simulink model "four_bots_CNN_DSM_7"  (R2018b)
settings: Solver=ode5  StartTime=0.0  StopTime=20.0  FixedStep=0.0002  RelTol=1e-3
(part 1 of 2)
settings Model: Creator=a1752760  LastModifiedBy=a1752760

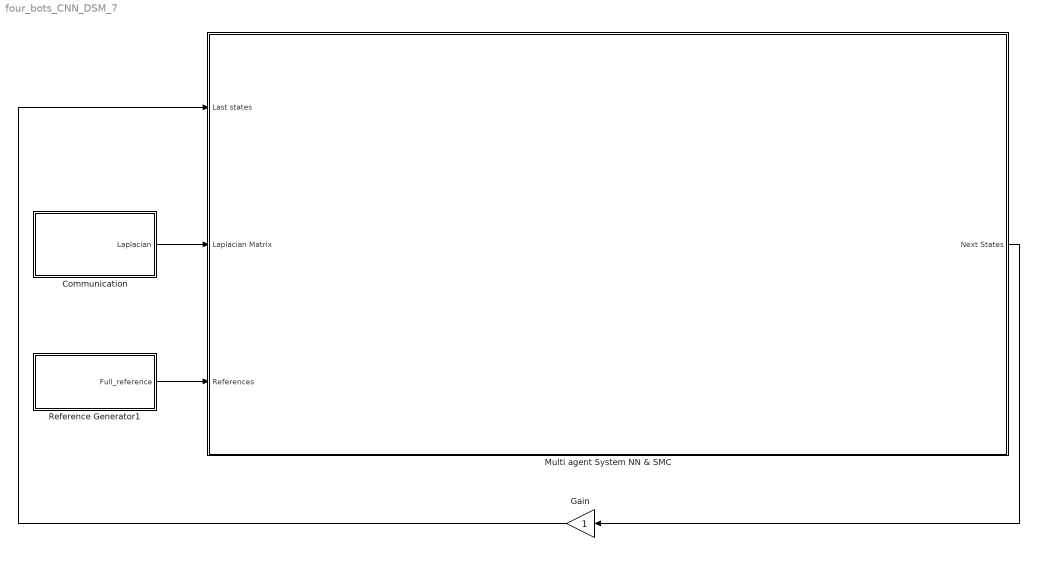
== system four_bots_CNN_DSM_7 ==
  Communication : Subsystem
  Gain : Gain
  Multi agent System NN & SMC : Subsystem
  Reference Generator1 : Subsystem
  wires:
  Multi agent System NN & SMC/1(Next States) -> Gain/1
  Communication/1(Laplacian) -> Multi agent System NN & SMC/2(Laplacian Matrix)
  Reference Generator1/1(Full_reference) -> Multi agent System NN & SMC/3("References ")
  Gain/1 -> Multi agent System NN & SMC/1(Last states)

== system four_bots_CNN_DSM_7/Communication ==
  Add : Sum
  Communication Topology : Constant  Value=[2,-1,0,-1;-1,2,-1,0;0,-1,2,-1;-1,0,-1,2]  VectorParams1D=off
  Constant : Constant  Value=2  VectorParams1D=off
  Product : Product
  Reference Feeding : Constant  Value=[1,0,0,0;0,1,0,0;0,0,1,0;0,0,0,1]  VectorParams1D=off
  Laplacian : Outport
  wires:
  Constant/1 -> Product/2
  Reference Feeding/1 -> Product/1
  Communication Topology/1 -> Add/1
  Product/1 -> Add/2
  Add/1 -> Laplacian/1

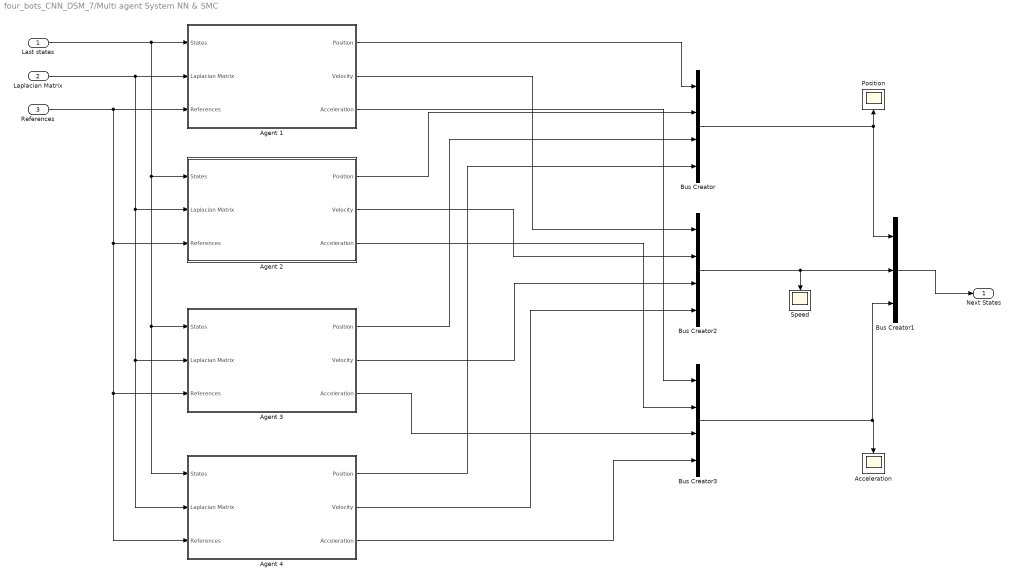
== system four_bots_CNN_DSM_7/Multi agent System NN & SMC ==
  Last states : Inport
  Laplacian Matrix : Inport  Port=2
  "References " : Inport  Port=3
  Acceleration : Scope
  "Agent 1 " : Subsystem
  Agent 2 : Subsystem
  Agent 3 : Subsystem
  Agent 4 : Subsystem
  Bus Creator : BusCreator  Inputs=4
  Bus Creator1 : BusCreator  Inputs=3
  Bus Creator2 : BusCreator  Inputs=4
  Bus Creator3 : BusCreator  Inputs=4
  Position : Scope
  Speed : Scope
  Next States : Outport
  wires:
  Bus Creator1/1 -> Next States/1
  Last states/1 -> Agent 4/1(States), Agent 3/1(States), Agent 2/1(States), "Agent 1 "/1(States)
  Laplacian Matrix/1 -> Agent 4/2(Laplacian Matrix), Agent 3/2(Laplacian Matrix), Agent 2/2(Laplacian Matrix), "Agent 1 "/2(Laplacian Matrix)
  "References "/1 -> Agent 4/3("References "), Agent 3/3("References "), Agent 2/3("References "), "Agent 1 "/3("References ")
  "Agent 1 "/1(Position) -> Bus Creator/1
  Agent 2/1(Position) -> Bus Creator/2
  Agent 3/1(Position) -> Bus Creator/3
  Agent 4/1(Position) -> Bus Creator/4
  "Agent 1 "/2(Velocity) -> Bus Creator2/1
  Agent 2/2(Velocity) -> Bus Creator2/2
  Agent 3/2(Velocity) -> Bus Creator2/3
  Agent 4/2(Velocity) -> Bus Creator2/4
  "Agent 1 "/3(Acceleration) -> Bus Creator3/1
  Agent 2/3(Acceleration) -> Bus Creator3/2
  Agent 3/3(Acceleration) -> Bus Creator3/3
  Agent 4/3(Acceleration) -> Bus Creator3/4
  Bus Creator/1 -> Bus Creator1/1, Position/1
  Bus Creator2/1 -> Speed/1, Bus Creator1/2
  Bus Creator3/1 -> Bus Creator1/3, Acceleration/1

== system four_bots_CNN_DSM_7/Reference Generator1 ==
  Acceleration reference : MATLAB Function  TreatAsAtomicUnit=on
  Acceleration_dot Reference : MATLAB Function  TreatAsAtomicUnit=on
  Acceleration_dot_ref : Scope
  Acceleration_ref : Scope
  Bus Creator1 : BusCreator  Inputs=4
  Clock : Clock
  Position Reference : MATLAB Function  TreatAsAtomicUnit=on
  Position_ref : Scope
  Speed Reference : MATLAB Function  TreatAsAtomicUnit=on
  Speed_ref : Scope
  Full_reference : Outport
  wires:
  Clock/1 -> Acceleration_dot Reference/1(t), Acceleration reference/1(t), Speed Reference/1(t), Position Reference/1(t)
  Position Reference/1(x1d) -> Position_ref/1, Bus Creator1/1
  Speed Reference/1(x2d) -> Speed_ref/1, Bus Creator1/2
  Acceleration reference/1(x2d_dot) -> Acceleration_ref/1, Bus Creator1/3
  Acceleration_dot Reference/1(x2ddot) -> Acceleration_dot_ref/1, Bus Creator1/4
  Bus Creator1/1 -> Full_reference/1

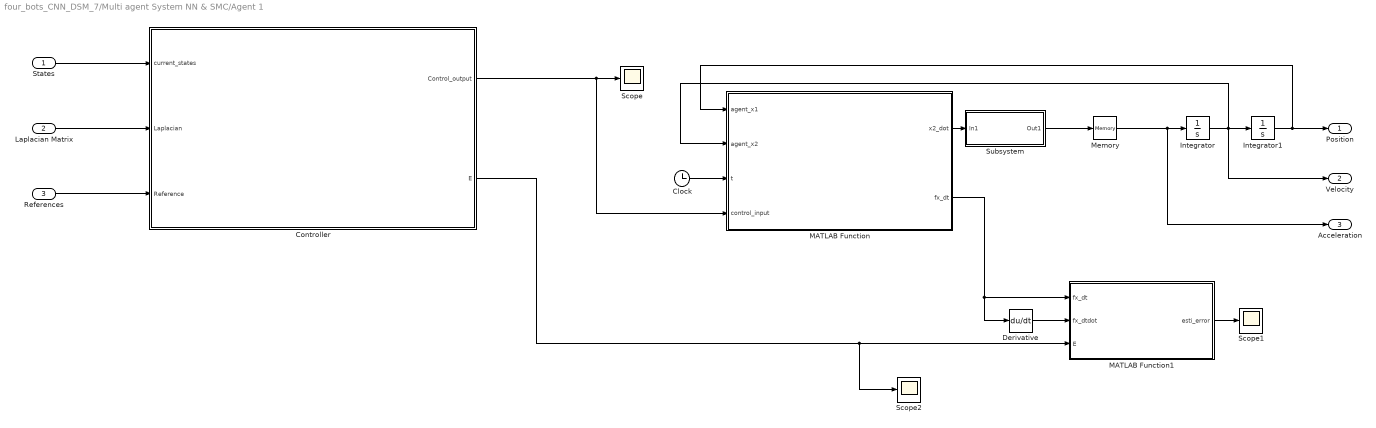
== system four_bots_CNN_DSM_7/Multi agent System NN & SMC/Agent 1  ==
  States : Inport
  Laplacian Matrix : Inport  Port=2
  "References " : Inport  Port=3
  Clock : Clock
  "Controller " : Subsystem
  Derivative : Derivative
  Integrator : Integrator  InitialCondition=[0;0;0]  ContinuousStateAttributes='speed'
  Integrator1 : Integrator  Tag=Position_x1  InitialCondition=[2;-1.5;-pi/3]  ContinuousStateAttributes='position'
  MATLAB Function : MATLAB Function  TreatAsAtomicUnit=on
  MATLAB Function1 : MATLAB Function  TreatAsAtomicUnit=on
  Memory : Memory  InitialCondition=[0;0;0]  LinearizeMemory=on
  Scope : Scope
  Scope1 : Scope
  Scope2 : Scope
  Subsystem : Subsystem
  Position : Outport
  Velocity : Outport  Port=2
  Acceleration : Outport  Port=3
  wires:
  MATLAB Function/2(fx_dt) -> MATLAB Function1/1(fx_dt), Derivative/1
  Integrator/1 -> Velocity/1, Integrator1/1, MATLAB Function/2(agent_x2)
  Integrator1/1 -> Position/1, MATLAB Function/1(agent_x1)
  MATLAB Function/1(x2_dot) -> Subsystem/1(In1)
  Subsystem/1(Out1) -> Memory/1
  States/1 -> "Controller "/1(current_states)
  Laplacian Matrix/1 -> "Controller "/2(Laplacian)
  "References "/1 -> "Controller "/3(Reference)
  "Controller "/1(Control_output) -> MATLAB Function/4(control_input), Scope/1
  Clock/1 -> MATLAB Function/3(t)
  Derivative/1 -> MATLAB Function1/2(fx_dtdot)
  "Controller "/2(E) -> Scope2/1, MATLAB Function1/3(E)
  MATLAB Function1/1(esti_error) -> Scope1/1
  Memory/1 -> Acceleration/1, Integrator/1

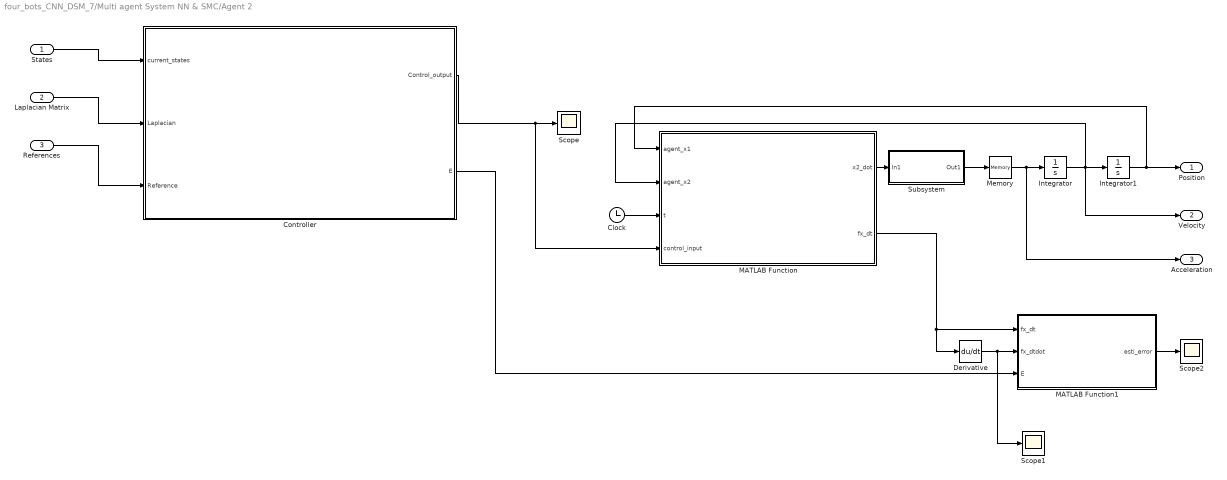
== system four_bots_CNN_DSM_7/Multi agent System NN & SMC/Agent 2 ==
  States : Inport
  Laplacian Matrix : Inport  Port=2
  "References " : Inport  Port=3
  Clock : Clock
  "Controller " : Subsystem
  Derivative : Derivative
  Integrator : Integrator  InitialCondition=[0;0;0]  ContinuousStateAttributes='speed'
  Integrator1 : Integrator  Tag=Position_x1  InitialCondition=[-1;1.5;pi/4]  ContinuousStateAttributes='position'
  MATLAB Function : MATLAB Function  TreatAsAtomicUnit=on
  MATLAB Function1 : MATLAB Function  TreatAsAtomicUnit=on
  Memory : Memory  InitialCondition=[0;0;0]  LinearizeMemory=on
  Scope : Scope
  Scope1 : Scope
  Scope2 : Scope
  Subsystem : Subsystem
  Position : Outport
  Velocity : Outport  Port=2
  Acceleration : Outport  Port=3
  wires:
  Integrator/1 -> Velocity/1, Integrator1/1, MATLAB Function/2(agent_x2)
  Integrator1/1 -> Position/1, MATLAB Function/1(agent_x1)
  MATLAB Function/1(x2_dot) -> Subsystem/1(In1)
  Subsystem/1(Out1) -> Memory/1
  States/1 -> "Controller "/1(current_states)
  Laplacian Matrix/1 -> "Controller "/2(Laplacian)
  "References "/1 -> "Controller "/3(Reference)
  "Controller "/1(Control_output) -> MATLAB Function/4(control_input), Scope/1
  "Controller "/2(E) -> MATLAB Function1/3(E)
  MATLAB Function1/1(esti_error) -> Scope2/1
  Derivative/1 -> Scope1/1, MATLAB Function1/2(fx_dtdot)
  MATLAB Function/2(fx_dt) -> MATLAB Function1/1(fx_dt), Derivative/1
  Clock/1 -> MATLAB Function/3(t)
  Memory/1 -> Acceleration/1, Integrator/1

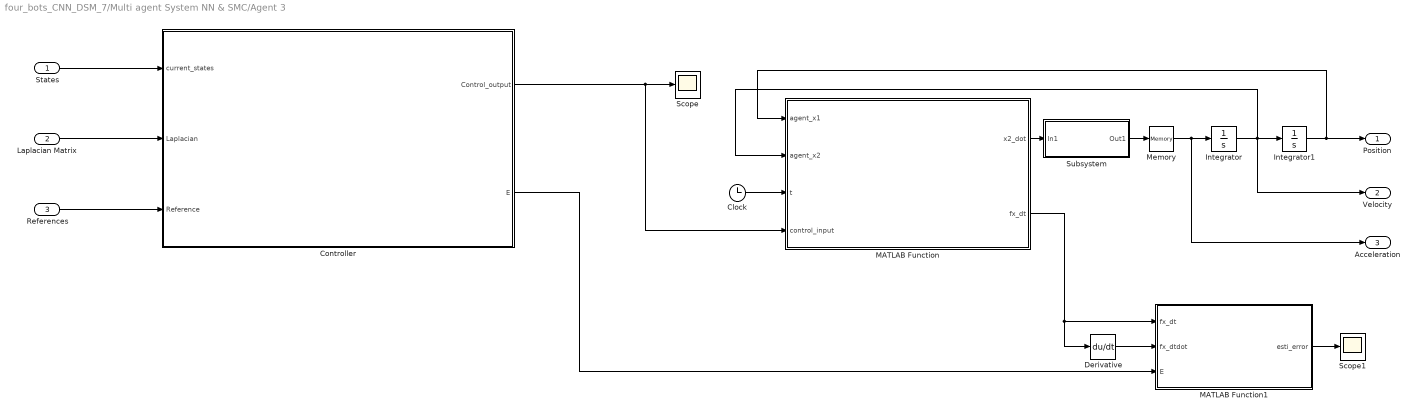
== system four_bots_CNN_DSM_7/Multi agent System NN & SMC/Agent 3 ==
  States : Inport
  Laplacian Matrix : Inport  Port=2
  "References " : Inport  Port=3
  Clock : Clock
  "Controller " : Subsystem
  Derivative : Derivative
  Integrator : Integrator  InitialCondition=[0;0;0]  ContinuousStateAttributes='speed'
  Integrator1 : Integrator  Tag=Position_x1  InitialCondition=[-3.5;1.5;-pi/6]  ContinuousStateAttributes='position'
  MATLAB Function : MATLAB Function  TreatAsAtomicUnit=on
  MATLAB Function1 : MATLAB Function  TreatAsAtomicUnit=on
  Memory : Memory  InitialCondition=[0;0;0]  LinearizeMemory=on
  Scope : Scope
  Scope1 : Scope
  Subsystem : Subsystem
  Position : Outport
  Velocity : Outport  Port=2
  Acceleration : Outport  Port=3
  wires:
  MATLAB Function/2(fx_dt) -> MATLAB Function1/1(fx_dt), Derivative/1
  Integrator/1 -> Velocity/1, Integrator1/1, MATLAB Function/2(agent_x2)
  Integrator1/1 -> Position/1, MATLAB Function/1(agent_x1)
  MATLAB Function/1(x2_dot) -> Subsystem/1(In1)
  Subsystem/1(Out1) -> Memory/1
  States/1 -> "Controller "/1(current_states)
  Laplacian Matrix/1 -> "Controller "/2(Laplacian)
  "References "/1 -> "Controller "/3(Reference)
  "Controller "/1(Control_output) -> MATLAB Function/4(control_input), Scope/1
  Clock/1 -> MATLAB Function/3(t)
  Derivative/1 -> MATLAB Function1/2(fx_dtdot)
  "Controller "/2(E) -> MATLAB Function1/3(E)
  MATLAB Function1/1(esti_error) -> Scope1/1
  Memory/1 -> Acceleration/1, Integrator/1

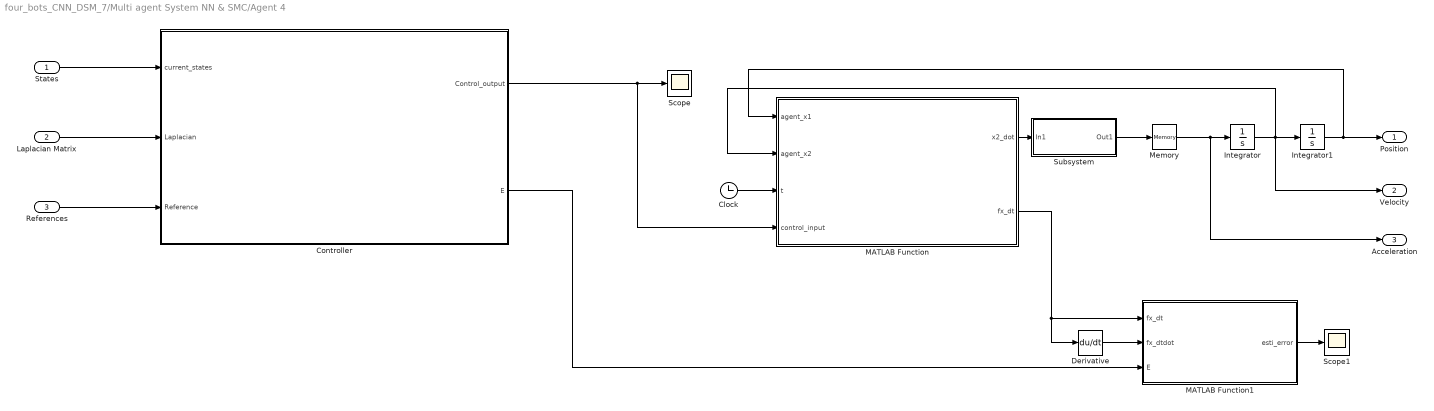
== system four_bots_CNN_DSM_7/Multi agent System NN & SMC/Agent 4 ==
  States : Inport
  Laplacian Matrix : Inport  Port=2
  "References " : Inport  Port=3
  Clock : Clock
  "Controller " : Subsystem
  Derivative : Derivative
  Integrator : Integrator  InitialCondition=[0;0;0]  ContinuousStateAttributes='speed'
  Integrator1 : Integrator  Tag=Position_x1  InitialCondition=[1.8;-3.3;pi/6]  ContinuousStateAttributes='position'
  MATLAB Function : MATLAB Function  TreatAsAtomicUnit=on
  MATLAB Function1 : MATLAB Function  TreatAsAtomicUnit=on
  Memory : Memory  InitialCondition=[0;0;0]  LinearizeMemory=on
  Scope : Scope
  Scope1 : Scope
  Subsystem : Subsystem
  Position : Outport
  Velocity : Outport  Port=2
  Acceleration : Outport  Port=3
  wires:
  MATLAB Function/2(fx_dt) -> MATLAB Function1/1(fx_dt), Derivative/1
  Integrator/1 -> Velocity/1, Integrator1/1, MATLAB Function/2(agent_x2)
  Integrator1/1 -> Position/1, MATLAB Function/1(agent_x1)
  MATLAB Function/1(x2_dot) -> Subsystem/1(In1)
  Subsystem/1(Out1) -> Memory/1
  States/1 -> "Controller "/1(current_states)
  Laplacian Matrix/1 -> "Controller "/2(Laplacian)
  "References "/1 -> "Controller "/3(Reference)
  "Controller "/1(Control_output) -> MATLAB Function/4(control_input), Scope/1
  Clock/1 -> MATLAB Function/3(t)
  Derivative/1 -> MATLAB Function1/2(fx_dtdot)
  "Controller "/2(E) -> MATLAB Function1/3(E)
  MATLAB Function1/1(esti_error) -> Scope1/1
  Memory/1 -> Acceleration/1, Integrator/1

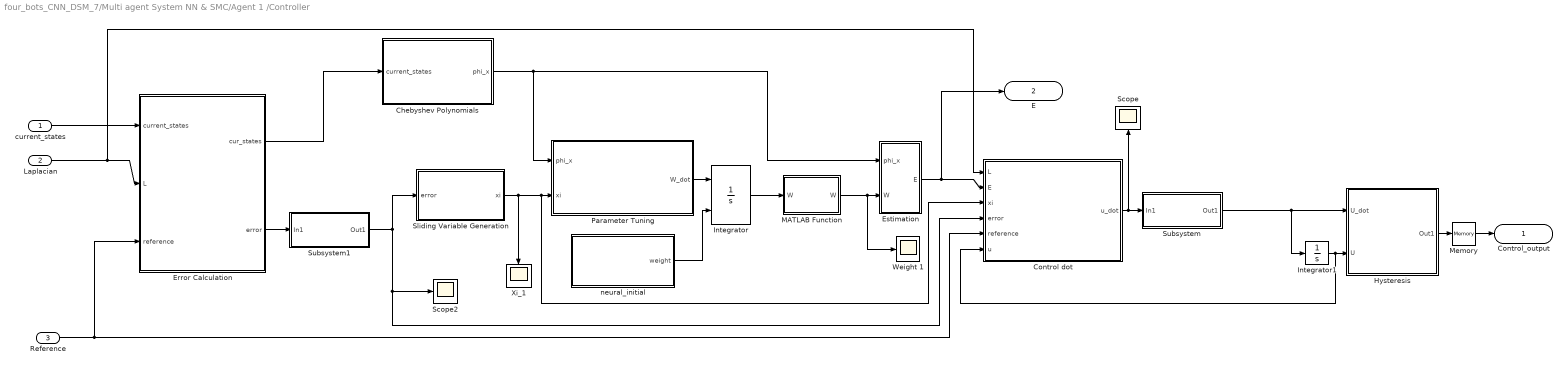
== system four_bots_CNN_DSM_7/Multi agent System NN & SMC/Agent 1 /Controller  ==
  current_states : Inport
  Laplacian : Inport  Port=2
  Reference : Inport  Port=3
  Chebyshev Polynomials : MATLAB Function  TreatAsAtomicUnit=on
  Control dot : MATLAB Function  TreatAsAtomicUnit=on
  Error Calculation : MATLAB Function  TreatAsAtomicUnit=on
  Estimation : MATLAB Function  TreatAsAtomicUnit=on
  Hysteresis : Subsystem
  Integrator : Integrator  InitialConditionSource=external  InitialCondition=[0 0 0]'  UpperSaturationLimit=200  LowerSaturationLimit=-200  ContinuousStateAttributes='Neural_weights'
  Integrator1 : Integrator  InitialCondition=[0;0;0]  UpperSaturationLimit=200  LowerSaturationLimit=-200  ContinuousStateAttributes='Control_output'
  MATLAB Function : MATLAB Function  TreatAsAtomicUnit=on
  Memory : Memory  InitialCondition=[0;0;0]  LinearizeMemory=on
  Parameter Tuning : MATLAB Function  TreatAsAtomicUnit=on
  Scope : Scope
  Scope2 : Scope
  Sliding Variable Generation : MATLAB Function  TreatAsAtomicUnit=on
  Subsystem : Subsystem
  Subsystem1 : Subsystem
  Weight 1 : Scope
  Xi_1 : Scope
  neural_initial : MATLAB Function  TreatAsAtomicUnit=on
  Control_output : Outport
  E : Outport  Port=2
  wires:
  current_states/1 -> Error Calculation/1(current_states)
  Reference/1 -> Error Calculation/3(reference), Control dot/5(reference)
  Sliding Variable Generation/1(xi) -> Xi_1/1, Control dot/3(xi), Parameter Tuning/2(xi)
  Chebyshev Polynomials/1(phi_x) -> Estimation/1(phi_x), Parameter Tuning/1(phi_x)
  Parameter Tuning/1(W_dot) -> Integrator/1
  neural_initial/1(weight) -> Integrator/2
  Integrator/1 -> MATLAB Function/1("W ")
  Estimation/1(E) -> E/1, Control dot/2(E)
  Control dot/1(u_dot) -> Subsystem/1(In1), Scope/1
  Error Calculation/2(error) -> Subsystem1/1(In1)
  Subsystem1/1(Out1) -> Sliding Variable Generation/1(error), Control dot/4(error), Scope2/1
  Integrator1/1 -> Hysteresis/2(U), Control dot/6(u)
  Laplacian/1 -> Control dot/1(L), Error Calculation/2(L)
  Error Calculation/1(cur_states) -> Chebyshev Polynomials/1(current_states)
  Hysteresis/1(Out1) -> Memory/1
  Subsystem/1(Out1) -> Integrator1/1, Hysteresis/1(U_dot)
  Memory/1 -> Control_output/1
  MATLAB Function/1(W) -> Weight 1/1, Estimation/2(W)

== system four_bots_CNN_DSM_7/Multi agent System NN & SMC/Agent 1 /Subsystem ==
  In1 : Inport
  Clock : Clock
  Constant : Constant  Value=[0;0;0]
  Scope3 : Scope
  Switch : Switch  Criteria=u2 > Threshold  Threshold=0.01
  Out1 : Outport
  wires:
  Constant/1 -> Switch/3
  In1/1 -> Switch/1
  Switch/1 -> Out1/1, Scope3/1
  Clock/1 -> Switch/2

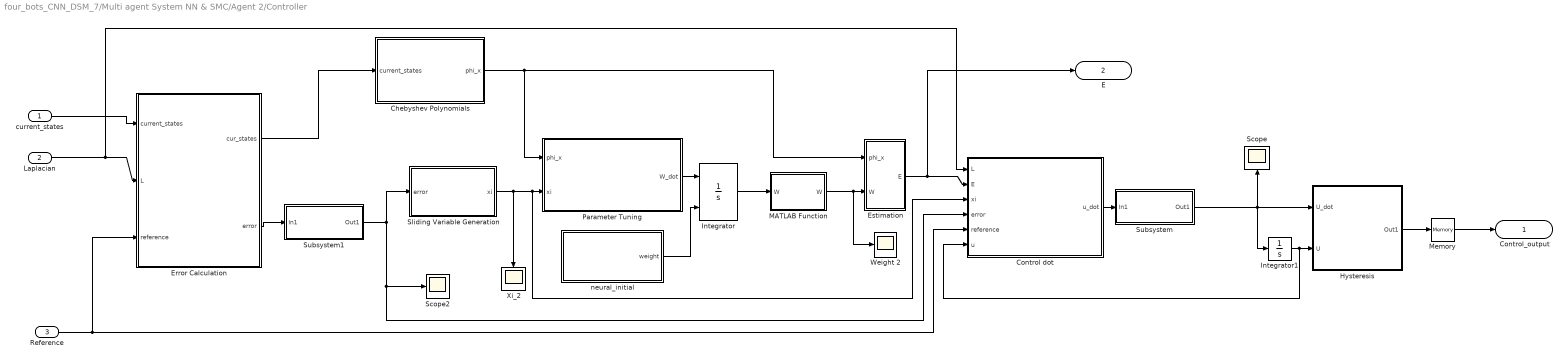
== system four_bots_CNN_DSM_7/Multi agent System NN & SMC/Agent 2/Controller  ==
  current_states : Inport
  Laplacian : Inport  Port=2
  Reference : Inport  Port=3
  Chebyshev Polynomials : MATLAB Function  TreatAsAtomicUnit=on
  Control dot : MATLAB Function  TreatAsAtomicUnit=on
  Error Calculation : MATLAB Function  TreatAsAtomicUnit=on
  Estimation : MATLAB Function  TreatAsAtomicUnit=on
  Hysteresis : Subsystem
  Integrator : Integrator  InitialConditionSource=external  InitialCondition=[0 0 0]'  UpperSaturationLimit=200  LowerSaturationLimit=-200  ContinuousStateAttributes='Neural_weights'
  Integrator1 : Integrator  InitialCondition=[0;0;0]  UpperSaturationLimit=200  LowerSaturationLimit=-200  ContinuousStateAttributes='Control_output'
  MATLAB Function : MATLAB Function  TreatAsAtomicUnit=on
  Memory : Memory  InitialCondition=[0;0;0]  LinearizeMemory=on
  Parameter Tuning : MATLAB Function  TreatAsAtomicUnit=on
  Scope : Scope
  Scope2 : Scope
  Sliding Variable Generation : MATLAB Function  TreatAsAtomicUnit=on
  Subsystem : Subsystem
  Subsystem1 : Subsystem
  Weight 2 : Scope
  Xi_2 : Scope
  neural_initial : MATLAB Function  TreatAsAtomicUnit=on
  Control_output : Outport
  E : Outport  Port=2
  wires:
  current_states/1 -> Error Calculation/1(current_states)
  Reference/1 -> Error Calculation/3(reference), Control dot/5(reference)
  Sliding Variable Generation/1(xi) -> Xi_2/1, Control dot/3(xi), Parameter Tuning/2(xi)
  Chebyshev Polynomials/1(phi_x) -> Estimation/1(phi_x), Parameter Tuning/1(phi_x)
  Parameter Tuning/1(W_dot) -> Integrator/1
  neural_initial/1(weight) -> Integrator/2
  Integrator/1 -> MATLAB Function/1("W ")
  Estimation/1(E) -> E/1, Control dot/2(E)
  Control dot/1(u_dot) -> Subsystem/1(In1)
  Error Calculation/2(error) -> Subsystem1/1(In1)
  Subsystem1/1(Out1) -> Sliding Variable Generation/1(error), Control dot/4(error), Scope2/1
  Integrator1/1 -> Hysteresis/2(U), Control dot/6(u)
  Laplacian/1 -> Control dot/1(L), Error Calculation/2(L)
  Error Calculation/1(cur_states) -> Chebyshev Polynomials/1(current_states)
  Hysteresis/1(Out1) -> Memory/1
  Subsystem/1(Out1) -> Integrator1/1, Scope/1, Hysteresis/1(U_dot)
  Memory/1 -> Control_output/1
  MATLAB Function/1(W) -> Weight 2/1, Estimation/2(W)

== system four_bots_CNN_DSM_7/Multi agent System NN & SMC/Agent 2/Subsystem ==
  In1 : Inport
  Clock : Clock
  Constant : Constant  Value=[0;0;0]
  Scope3 : Scope
  Switch : Switch  Criteria=u2 > Threshold  Threshold=0.01
  Out1 : Outport
  wires:
  Constant/1 -> Switch/3
  In1/1 -> Switch/1
  Switch/1 -> Out1/1, Scope3/1
  Clock/1 -> Switch/2

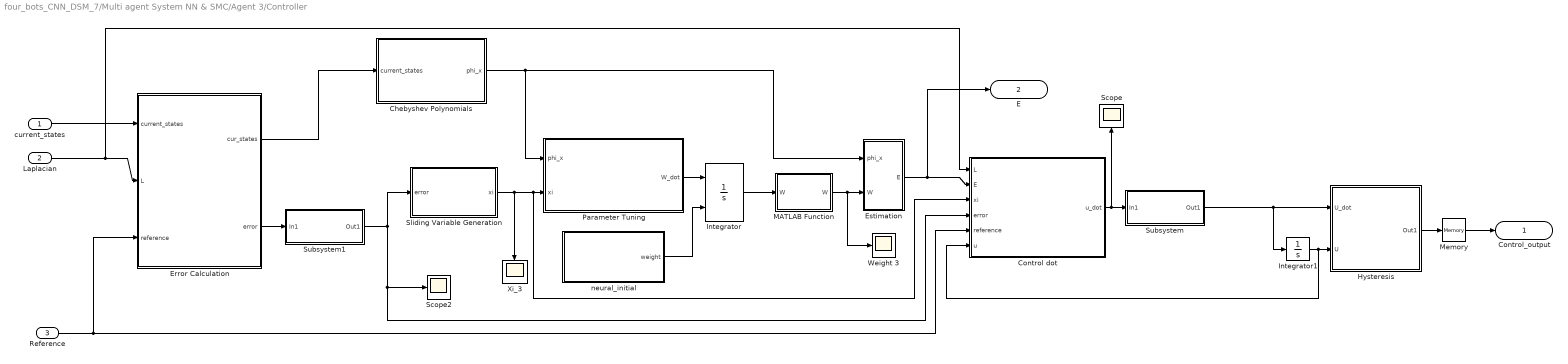
== system four_bots_CNN_DSM_7/Multi agent System NN & SMC/Agent 3/Controller  ==
  current_states : Inport
  Laplacian : Inport  Port=2
  Reference : Inport  Port=3
  Chebyshev Polynomials : MATLAB Function  TreatAsAtomicUnit=on
  Control dot : MATLAB Function  TreatAsAtomicUnit=on
  Error Calculation : MATLAB Function  TreatAsAtomicUnit=on
  Estimation : MATLAB Function  TreatAsAtomicUnit=on
  Hysteresis : Subsystem
  Integrator : Integrator  InitialConditionSource=external  InitialCondition=[0 0 0]'  UpperSaturationLimit=200  LowerSaturationLimit=-200  ContinuousStateAttributes='Neural_weights'
  Integrator1 : Integrator  InitialCondition=[0;0;0]  UpperSaturationLimit=200  LowerSaturationLimit=-200  ContinuousStateAttributes='Control_output'
  MATLAB Function : MATLAB Function  TreatAsAtomicUnit=on
  Memory : Memory  InitialCondition=[0;0;0]  LinearizeMemory=on
  Parameter Tuning : MATLAB Function  TreatAsAtomicUnit=on
  Scope : Scope
  Scope2 : Scope
  Sliding Variable Generation : MATLAB Function  TreatAsAtomicUnit=on
  Subsystem : Subsystem
  Subsystem1 : Subsystem
  Weight 3 : Scope
  Xi_3 : Scope
  neural_initial : MATLAB Function  TreatAsAtomicUnit=on
  Control_output : Outport
  E : Outport  Port=2
  wires:
  current_states/1 -> Error Calculation/1(current_states)
  Reference/1 -> Error Calculation/3(reference), Control dot/5(reference)
  Sliding Variable Generation/1(xi) -> Xi_3/1, Control dot/3(xi), Parameter Tuning/2(xi)
  Chebyshev Polynomials/1(phi_x) -> Estimation/1(phi_x), Parameter Tuning/1(phi_x)
  Parameter Tuning/1(W_dot) -> Integrator/1
  neural_initial/1(weight) -> Integrator/2
  Integrator/1 -> MATLAB Function/1("W ")
  Estimation/1(E) -> E/1, Control dot/2(E)
  Control dot/1(u_dot) -> Subsystem/1(In1), Scope/1
  Error Calculation/2(error) -> Subsystem1/1(In1)
  Subsystem1/1(Out1) -> Sliding Variable Generation/1(error), Control dot/4(error), Scope2/1
  Integrator1/1 -> Hysteresis/2(U), Control dot/6(u)
  Laplacian/1 -> Control dot/1(L), Error Calculation/2(L)
  Error Calculation/1(cur_states) -> Chebyshev Polynomials/1(current_states)
  Hysteresis/1(Out1) -> Memory/1
  Subsystem/1(Out1) -> Hysteresis/1(U_dot), Integrator1/1
  Memory/1 -> Control_output/1
  MATLAB Function/1(W) -> Estimation/2(W), Weight 3/1

== system four_bots_CNN_DSM_7/Multi agent System NN & SMC/Agent 3/Subsystem ==
  In1 : Inport
  Clock : Clock
  Constant : Constant  Value=[0;0;0]
  Scope3 : Scope
  Switch : Switch  Criteria=u2 > Threshold  Threshold=0.01
  Out1 : Outport
  wires:
  Constant/1 -> Switch/3
  In1/1 -> Switch/1
  Switch/1 -> Out1/1, Scope3/1
  Clock/1 -> Switch/2

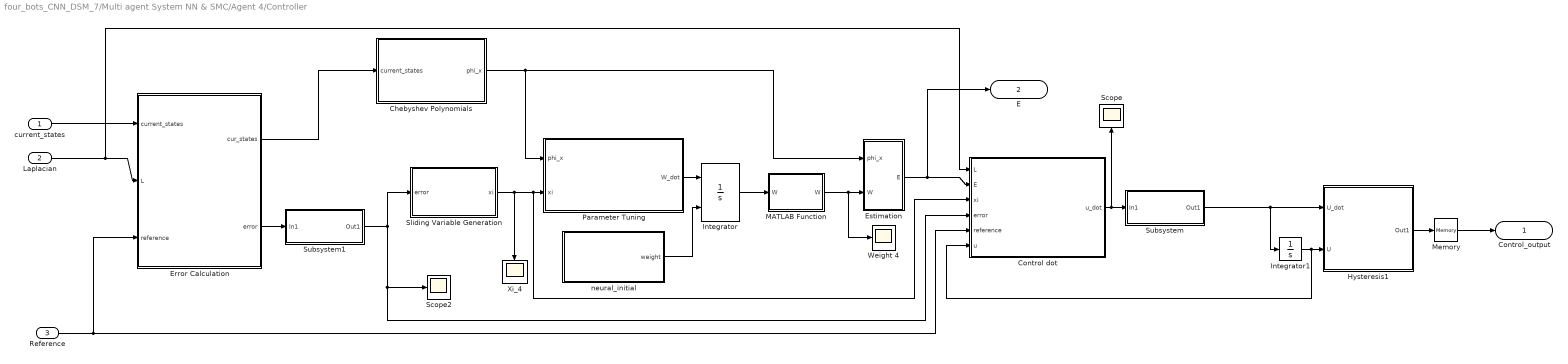
== system four_bots_CNN_DSM_7/Multi agent System NN & SMC/Agent 4/Controller  ==
  current_states : Inport
  Laplacian : Inport  Port=2
  Reference : Inport  Port=3
  Chebyshev Polynomials : MATLAB Function  TreatAsAtomicUnit=on
  Control dot : MATLAB Function  TreatAsAtomicUnit=on
  Error Calculation : MATLAB Function  TreatAsAtomicUnit=on
  Estimation : MATLAB Function  TreatAsAtomicUnit=on
  Hysteresis1 : Subsystem
  Integrator : Integrator  InitialConditionSource=external  InitialCondition=[0 0 0]'  UpperSaturationLimit=200  LowerSaturationLimit=-200  ContinuousStateAttributes='Neural_weights'
  Integrator1 : Integrator  InitialCondition=[0;0;0]  UpperSaturationLimit=200  LowerSaturationLimit=-200  ContinuousStateAttributes='Control_output'
  MATLAB Function : MATLAB Function  TreatAsAtomicUnit=on
  Memory : Memory  InitialCondition=[0;0;0]  LinearizeMemory=on
  Parameter Tuning : MATLAB Function  TreatAsAtomicUnit=on
  Scope : Scope
  Scope2 : Scope
  Sliding Variable Generation : MATLAB Function  TreatAsAtomicUnit=on
  Subsystem : Subsystem
  Subsystem1 : Subsystem
  Weight 4 : Scope
  Xi_4 : Scope
  neural_initial : MATLAB Function  TreatAsAtomicUnit=on
  Control_output : Outport
  E : Outport  Port=2
  wires:
  current_states/1 -> Error Calculation/1(current_states)
  Reference/1 -> Error Calculation/3(reference), Control dot/5(reference)
  Sliding Variable Generation/1(xi) -> Xi_4/1, Control dot/3(xi), Parameter Tuning/2(xi)
  Chebyshev Polynomials/1(phi_x) -> Estimation/1(phi_x), Parameter Tuning/1(phi_x)
  Parameter Tuning/1(W_dot) -> Integrator/1
  neural_initial/1(weight) -> Integrator/2
  Integrator/1 -> MATLAB Function/1("W ")
  Estimation/1(E) -> E/1, Control dot/2(E)
  Control dot/1(u_dot) -> Subsystem/1(In1), Scope/1
  Error Calculation/2(error) -> Subsystem1/1(In1)
  Subsystem1/1(Out1) -> Sliding Variable Generation/1(error), Control dot/4(error), Scope2/1
  Integrator1/1 -> Hysteresis1/2(U), Control dot/6(u)
  Laplacian/1 -> Control dot/1(L), Error Calculation/2(L)
  Error Calculation/1(cur_states) -> Chebyshev Polynomials/1(current_states)
  Hysteresis1/1(Out1) -> Memory/1
  Subsystem/1(Out1) -> Hysteresis1/1(U_dot), Integrator1/1
  Memory/1 -> Control_output/1
  MATLAB Function/1(W) -> Estimation/2(W), Weight 4/1

== system four_bots_CNN_DSM_7/Multi agent System NN & SMC/Agent 4/Subsystem ==
  In1 : Inport
  Clock : Clock
  Constant : Constant  Value=[0;0;0]
  Scope3 : Scope
  Switch : Switch  Criteria=u2 > Threshold  Threshold=0.01
  Out1 : Outport
  wires:
  Constant/1 -> Switch/3
  In1/1 -> Switch/1
  Switch/1 -> Out1/1, Scope3/1
  Clock/1 -> Switch/2

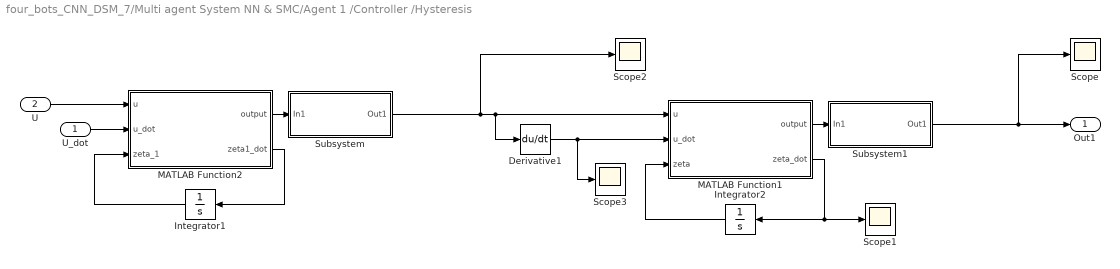
== system four_bots_CNN_DSM_7/Multi agent System NN & SMC/Agent 1 /Controller /Hysteresis ==
  U_dot : Inport
  U : Inport  Port=2
  Derivative1 : Derivative
  Integrator1 : Integrator  InitialCondition=[0;0;0]  ContinuousStateAttributes='speed'
  Integrator2 : Integrator  InitialCondition=[0;0;0]  ContinuousStateAttributes='speed'
  MATLAB Function1 : MATLAB Function  TreatAsAtomicUnit=on
  MATLAB Function2 : MATLAB Function  TreatAsAtomicUnit=on
  Scope{,1..3} (4 alike) : Scope
  Subsystem : Subsystem
  Subsystem1 : Subsystem
  Out1 : Outport
  wires:
  Integrator1/1 -> MATLAB Function2/3(zeta_1)
  MATLAB Function2/2(zeta1_dot) -> Integrator1/1
  U/1 -> MATLAB Function2/1(u)
  U_dot/1 -> MATLAB Function2/2(u_dot)
  Derivative1/1 -> Scope3/1, MATLAB Function1/2(u_dot)
  Integrator2/1 -> MATLAB Function1/3(zeta)
  MATLAB Function1/2(zeta_dot) -> Integrator2/1, Scope1/1
  MATLAB Function2/1(output) -> Subsystem/1(In1)
  MATLAB Function1/1(output) -> Subsystem1/1(In1)
  Subsystem/1(Out1) -> Scope2/1, Derivative1/1, MATLAB Function1/1(u)
  Subsystem1/1(Out1) -> Scope/1, Out1/1

== system four_bots_CNN_DSM_7/Multi agent System NN & SMC/Agent 1 /Controller /Subsystem ==
  In1 : Inport
  Clock : Clock
  Constant : Constant  Value=[0;0;0]
  Scope3 : Scope
  Switch : Switch  Criteria=u2 > Threshold  Threshold=0.01
  Out1 : Outport
  wires:
  Constant/1 -> Switch/3
  In1/1 -> Switch/1
  Switch/1 -> Out1/1, Scope3/1
  Clock/1 -> Switch/2

== system four_bots_CNN_DSM_7/Multi agent System NN & SMC/Agent 1 /Controller /Subsystem1 ==
  In1 : Inport
  Clock : Clock
  Constant : Constant  Value=zeros(9,1)
  Scope3 : Scope
  Switch : Switch  Criteria=u2 > Threshold  Threshold=0.01
  Out1 : Outport
  wires:
  Constant/1 -> Switch/3
  In1/1 -> Switch/1
  Switch/1 -> Out1/1, Scope3/1
  Clock/1 -> Switch/2

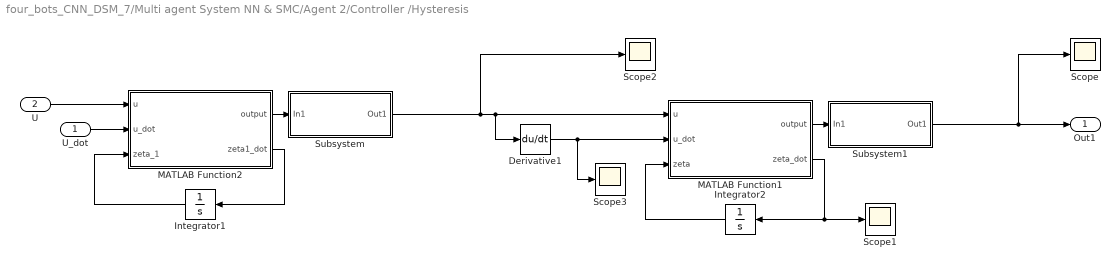
== system four_bots_CNN_DSM_7/Multi agent System NN & SMC/Agent 2/Controller /Hysteresis ==
  U_dot : Inport
  U : Inport  Port=2
  Derivative1 : Derivative
  Integrator1 : Integrator  InitialCondition=[0;0;0]  ContinuousStateAttributes='speed'
  Integrator2 : Integrator  InitialCondition=[0;0;0]  ContinuousStateAttributes='speed'
  MATLAB Function1 : MATLAB Function  TreatAsAtomicUnit=on
  MATLAB Function2 : MATLAB Function  TreatAsAtomicUnit=on
  Scope{,1..3} (4 alike) : Scope
  Subsystem : Subsystem
  Subsystem1 : Subsystem
  Out1 : Outport
  wires:
  Integrator1/1 -> MATLAB Function2/3(zeta_1)
  MATLAB Function2/2(zeta1_dot) -> Integrator1/1
  U/1 -> MATLAB Function2/1(u)
  U_dot/1 -> MATLAB Function2/2(u_dot)
  Derivative1/1 -> Scope3/1, MATLAB Function1/2(u_dot)
  Integrator2/1 -> MATLAB Function1/3(zeta)
  MATLAB Function1/2(zeta_dot) -> Integrator2/1, Scope1/1
  MATLAB Function2/1(output) -> Subsystem/1(In1)
  MATLAB Function1/1(output) -> Subsystem1/1(In1)
  Subsystem/1(Out1) -> Scope2/1, Derivative1/1, MATLAB Function1/1(u)
  Subsystem1/1(Out1) -> Out1/1, Scope/1

== system four_bots_CNN_DSM_7/Multi agent System NN & SMC/Agent 2/Controller /Subsystem ==
  In1 : Inport
  Clock : Clock
  Constant : Constant  Value=[0;0;0]
  Scope3 : Scope
  Switch : Switch  Criteria=u2 > Threshold  Threshold=0.01
  Out1 : Outport
  wires:
  Constant/1 -> Switch/3
  In1/1 -> Switch/1
  Switch/1 -> Out1/1, Scope3/1
  Clock/1 -> Switch/2

== system four_bots_CNN_DSM_7/Multi agent System NN & SMC/Agent 2/Controller /Subsystem1 ==
  In1 : Inport
  Clock : Clock
  Constant : Constant  Value=zeros(9,1)
  Scope3 : Scope
  Switch : Switch  Criteria=u2 > Threshold  Threshold=0.01
  Out1 : Outport
  wires:
  Constant/1 -> Switch/3
  In1/1 -> Switch/1
  Switch/1 -> Out1/1, Scope3/1
  Clock/1 -> Switch/2

== system four_bots_CNN_DSM_7/Multi agent System NN & SMC/Agent 3/Controller /Hysteresis ==
  U_dot : Inport
  U : Inport  Port=2
  Derivative1 : Derivative
  Integrator1 : Integrator  InitialCondition=[0;0;0]  ContinuousStateAttributes='speed'
  Integrator2 : Integrator  InitialCondition=[0;0;0]  ContinuousStateAttributes='speed'
  MATLAB Function1 : MATLAB Function  TreatAsAtomicUnit=on
  MATLAB Function2 : MATLAB Function  TreatAsAtomicUnit=on
  Scope{,1..3} (4 alike) : Scope
  Subsystem : Subsystem
  Subsystem1 : Subsystem
  Out1 : Outport
  wires:
  Integrator1/1 -> MATLAB Function2/3(zeta_1)
  MATLAB Function2/2(zeta1_dot) -> Integrator1/1
  U/1 -> MATLAB Function2/1(u)
  U_dot/1 -> MATLAB Function2/2(u_dot)
  Derivative1/1 -> Scope3/1, MATLAB Function1/2(u_dot)
  Integrator2/1 -> MATLAB Function1/3(zeta)
  MATLAB Function1/2(zeta_dot) -> Integrator2/1, Scope1/1
  MATLAB Function2/1(output) -> Subsystem/1(In1)
  MATLAB Function1/1(output) -> Subsystem1/1(In1)
  Subsystem/1(Out1) -> Scope2/1, Derivative1/1, MATLAB Function1/1(u)
  Subsystem1/1(Out1) -> Out1/1, Scope/1

== system four_bots_CNN_DSM_7/Multi agent System NN & SMC/Agent 3/Controller /Subsystem ==
  In1 : Inport
  Clock : Clock
  Constant : Constant  Value=[0;0;0]
  Scope3 : Scope
  Switch : Switch  Criteria=u2 > Threshold  Threshold=0.01
  Out1 : Outport
  wires:
  Constant/1 -> Switch/3
  In1/1 -> Switch/1
  Switch/1 -> Out1/1, Scope3/1
  Clock/1 -> Switch/2

== system four_bots_CNN_DSM_7/Multi agent System NN & SMC/Agent 3/Controller /Subsystem1 ==
  In1 : Inport
  Clock : Clock
  Constant : Constant  Value=zeros(9,1)
  Scope3 : Scope
  Switch : Switch  Criteria=u2 > Threshold  Threshold=0.01
  Out1 : Outport
  wires:
  Constant/1 -> Switch/3
  In1/1 -> Switch/1
  Switch/1 -> Out1/1, Scope3/1
  Clock/1 -> Switch/2

== system four_bots_CNN_DSM_7/Multi agent System NN & SMC/Agent 4/Controller /Hysteresis1 ==
  U_dot : Inport
  U : Inport  Port=2
  Derivative1 : Derivative
  Integrator1 : Integrator  InitialCondition=[0;0;0]  ContinuousStateAttributes='speed'
  Integrator2 : Integrator  InitialCondition=[0;0;0]  ContinuousStateAttributes='speed'
  MATLAB Function1 : MATLAB Function  TreatAsAtomicUnit=on
  MATLAB Function2 : MATLAB Function  TreatAsAtomicUnit=on
  Scope{,1..3} (4 alike) : Scope
  Subsystem : Subsystem
  Subsystem1 : Subsystem
  Out1 : Outport
  wires:
  Integrator1/1 -> MATLAB Function2/3(zeta_1)
  MATLAB Function2/2(zeta1_dot) -> Integrator1/1
  U/1 -> MATLAB Function2/1(u)
  U_dot/1 -> MATLAB Function2/2(u_dot)
  Derivative1/1 -> Scope3/1, MATLAB Function1/2(u_dot)
  Integrator2/1 -> MATLAB Function1/3(zeta)
  MATLAB Function1/2(zeta_dot) -> Integrator2/1, Scope1/1
  MATLAB Function2/1(output) -> Subsystem/1(In1)
  MATLAB Function1/1(output) -> Subsystem1/1(In1)
  Subsystem/1(Out1) -> Scope2/1, Derivative1/1, MATLAB Function1/1(u)
  Subsystem1/1(Out1) -> Out1/1, Scope/1

== system four_bots_CNN_DSM_7/Multi agent System NN & SMC/Agent 4/Controller /Subsystem ==
  In1 : Inport
  Clock : Clock
  Constant : Constant  Value=[0;0;0]
  Scope3 : Scope
  Switch : Switch  Criteria=u2 > Threshold  Threshold=0.01
  Out1 : Outport
  wires:
  Constant/1 -> Switch/3
  In1/1 -> Switch/1
  Switch/1 -> Out1/1, Scope3/1
  Clock/1 -> Switch/2

== system four_bots_CNN_DSM_7/Multi agent System NN & SMC/Agent 4/Controller /Subsystem1 ==
  In1 : Inport
  Clock : Clock
  Constant : Constant  Value=zeros(9,1)
  Scope3 : Scope
  Switch : Switch  Criteria=u2 > Threshold  Threshold=0.01
  Out1 : Outport
  wires:
  Constant/1 -> Switch/3
  In1/1 -> Switch/1
  Switch/1 -> Out1/1, Scope3/1
  Clock/1 -> Switch/2

== system four_bots_CNN_DSM_7/Multi agent System NN & SMC/Agent 1 /Controller /Hysteresis/Subsystem ==
  In1 : Inport
  Clock : Clock
  Constant : Constant  Value=[0;0;0]
  Scope3 : Scope
  Switch : Switch  Criteria=u2 > Threshold  Threshold=0.01
  Out1 : Outport
  wires:
  Constant/1 -> Switch/3
  In1/1 -> Switch/1
  Switch/1 -> Out1/1, Scope3/1
  Clock/1 -> Switch/2

== system four_bots_CNN_DSM_7/Multi agent System NN & SMC/Agent 1 /Controller /Hysteresis/Subsystem1 ==
  In1 : Inport
  Clock : Clock
  Constant : Constant  Value=[0;0;0]
  Scope3 : Scope
  Switch : Switch  Criteria=u2 > Threshold  Threshold=0.01
  Out1 : Outport
  wires:
  Constant/1 -> Switch/3
  In1/1 -> Switch/1
  Switch/1 -> Out1/1, Scope3/1
  Clock/1 -> Switch/2

== system four_bots_CNN_DSM_7/Multi agent System NN & SMC/Agent 2/Controller /Hysteresis/Subsystem ==
  In1 : Inport
  Clock : Clock
  Constant : Constant  Value=[0;0;0]
  Scope3 : Scope
  Switch : Switch  Criteria=u2 > Threshold  Threshold=0.01
  Out1 : Outport
  wires:
  Constant/1 -> Switch/3
  In1/1 -> Switch/1
  Switch/1 -> Out1/1, Scope3/1
  Clock/1 -> Switch/2

== system four_bots_CNN_DSM_7/Multi agent System NN & SMC/Agent 2/Controller /Hysteresis/Subsystem1 ==
  In1 : Inport
  Clock : Clock
  Constant : Constant  Value=[0;0;0]
  Scope3 : Scope
  Switch : Switch  Criteria=u2 > Threshold  Threshold=0.01
  Out1 : Outport
  wires:
  Constant/1 -> Switch/3
  In1/1 -> Switch/1
  Switch/1 -> Out1/1, Scope3/1
  Clock/1 -> Switch/2

== system four_bots_CNN_DSM_7/Multi agent System NN & SMC/Agent 3/Controller /Hysteresis/Subsystem ==
  In1 : Inport
  Clock : Clock
  Constant : Constant  Value=[0;0;0]
  Scope3 : Scope
  Switch : Switch  Criteria=u2 > Threshold  Threshold=0.01
  Out1 : Outport
  wires:
  Constant/1 -> Switch/3
  In1/1 -> Switch/1
  Switch/1 -> Out1/1, Scope3/1
  Clock/1 -> Switch/2

== system four_bots_CNN_DSM_7/Multi agent System NN & SMC/Agent 3/Controller /Hysteresis/Subsystem1 ==
  In1 : Inport
  Clock : Clock
  Constant : Constant  Value=[0;0;0]
  Scope3 : Scope
  Switch : Switch  Criteria=u2 > Threshold  Threshold=0.01
  Out1 : Outport
  wires:
  Constant/1 -> Switch/3
  In1/1 -> Switch/1
  Switch/1 -> Out1/1, Scope3/1
  Clock/1 -> Switch/2

== system four_bots_CNN_DSM_7/Multi agent System NN & SMC/Agent 4/Controller /Hysteresis1/Subsystem ==
  In1 : Inport
  Clock : Clock
  Constant : Constant  Value=[0;0;0]
  Scope3 : Scope
  Switch : Switch  Criteria=u2 > Threshold  Threshold=0.01
  Out1 : Outport
  wires:
  Constant/1 -> Switch/3
  In1/1 -> Switch/1
  Switch/1 -> Out1/1, Scope3/1
  Clock/1 -> Switch/2

== system four_bots_CNN_DSM_7/Multi agent System NN & SMC/Agent 4/Controller /Hysteresis1/Subsystem1 ==
  In1 : Inport
  Clock : Clock
  Constant : Constant  Value=[0;0;0]
  Scope3 : Scope
  Switch : Switch  Criteria=u2 > Threshold  Threshold=0.01
  Out1 : Outport
  wires:
  Constant/1 -> Switch/3
  In1/1 -> Switch/1
  Switch/1 -> Out1/1, Scope3/1
  Clock/1 -> Switch/2

== matlab function four_bots_CNN_DSM_7/Multi agent System NN & SMC/Agent 1 /Controller /Chebyshev Polynomials ==
  data: current_states input; phi_x output
function phi_x = Chebyshev_polynomials(current_states)

%% parameters that may alter
dimension=3;
cheby_order=3;

%% current states
x1=current_states(dimension*0+1:dimension*1);
x2=current_states(dimension*1+1:dimension*2);

%% initialization
phi_x=ones(1+2*dimension*cheby_order,1);

%% recursion procedure
now_x=[x1;x2];
for order = 1 : cheby_order
   if order == 1
      phi_x(2*dimension*(order-1)+2:2*dimension*order+1)=now_x;
   elseif order == 2
      phi_x(2*dimension*(order-1)+2:2*dimension*order+1)=2*now_x.*phi_x(2*dimension*(order-2)+2:2*dimension*(order-1)+1)-1;
   else
      phi_x(2*dimension*(order-1)+2:2*dimension*order+1)=2*now_x.*phi_x(2*dimension*(order-2)+2:2*dimension*(order-1)+1)-phi_x(2*dimension*(order-3)+2:2*dimension*(order-2)+1);
   end
end

end

== matlab function four_bots_CNN_DSM_7/Multi agent System NN & SMC/Agent 1 /MATLAB Function ==
  data: agent_x1 input; x2_dot output; agent_x2 input; t input; control_input input; fx_dt output
function [x2_dot, fx_dt] = physical_model( agent_x1 , agent_x2, t, control_input )

Mass=[4,5,4,5];
Alpha=[0.087,0.090,0.085,0.092];
Radius=[0.18,0.20,0.24,0.22];
Inertia=[0.12,0.15,0.13,0.14];
Beta=[11.4,11.6,11.8,12.0];

%% assign the parameter according to serial number
serial_num = 1; 
m=Mass(serial_num);
alpha=Alpha(serial_num);
R=Radius(serial_num);
inertia=Inertia(serial_num);
beta=Beta(serial_num);

%% current states of the robot
dimension=3;

theta=agent_x1(dimension);

%% the real model of robot
M=diag([1/m,1/m,1/inertia]);
T=[-sin(theta), -sin(pi/3-theta), sin(pi/3+theta);
    cos(theta), -cos(pi/3-theta), -cos(pi/3+theta);
    R,          R,                  R];

real_fx = -beta*M*(T*T')*agent_x2;
uncertain = [0.3*sin(0.5*t)+2; 0.2*cos(0.5*t)+1.5; 0.1*sin(0.3*t)+1];

%% saturation is added here for convinience
Vmax=6; % the maximum voltage of the motor

u1up=Vmax/(alpha*m)*(abs(sin(theta))+abs(sin(pi/3-theta))+abs(sin(pi/3+theta)));
u1do=-Vmax/(alpha*m)*(abs(sin(theta))+abs(sin(pi/3-theta))+abs(sin(pi/3+theta)));
u2up=Vmax/(alpha*m)*(abs(cos(theta))+abs(cos(pi/3-theta))+abs(cos(pi/3+theta)));
u2do=-Vmax/(alpha*m)*(abs(cos(theta))+abs(cos(pi/3-theta))+abs(cos(pi/3+theta)));
u3up=R/(alpha*inertia)*3*Vmax;
u3do=-R/(alpha*inertia)*3*Vmax;

control_input(1) = max( min(control_input(1),u1up), u1do );
control_input(2) = max( min(control_input(2),u2up), u2do );
control_input(3) = max( min(control_input(3),u3up), u3do );


fx_dt=real_fx + uncertain; 

x2_dot = real_fx + control_input + uncertain;


end

== matlab function four_bots_CNN_DSM_7/Multi agent System NN & SMC/Agent 1 /Controller /Error Calculation ==
  data: cur_states output; current_states input; L input; error output; reference input
function [cur_states , error] = error_calculation(current_states, L, reference)

%% parameters that may change for alternative use
dimension=3;
serial_num=1;

num_agent=size(L,1);
%% current states
% get current states
pos=current_states(dimension*num_agent*0+1 : dimension*num_agent*1);
vol=current_states(dimension*num_agent*1+1 : dimension*num_agent*2);
acc=current_states(dimension*num_agent*2+1 : dimension*num_agent*3);

% get current reference
r_pos=reference(dimension*num_agent*0+1 : dimension*num_agent*1);
r_vol=reference(dimension*num_agent*1+1 : dimension*num_agent*2);
r_acc=reference(dimension*num_agent*2+1 : dimension*num_agent*3);

% agent j's states
agent_x1 = pos(dimension*(serial_num-1)+1 : dimension*serial_num);
agent_x2 = vol(dimension*(serial_num-1)+1 : dimension*serial_num);

% agent_x2dot = acc(dimension*(serial_num-1)+1 : dimension*serial_num);
% 
% % agent j's reference
% r_x1=r_pos(dimension*(serial_num-1)+1 : dimension*serial_num);
% r_x2=r_vol(dimension*(serial_num-1)+1 : dimension*serial_num);
% r_x2dot=r_acc(dimension*(serial_num-1)+1 : dimension*serial_num);

e_1 = kron(L(serial_num, : ), eye(dimension) ) * (pos - r_pos);
e_2 = kron(L(serial_num, : ), eye(dimension) ) * (vol - r_vol);
e_2dot = kron(L(serial_num, : ), eye(dimension) ) * (acc - r_acc);

cur_states = [agent_x1;agent_x2];
error = [e_1 ; e_2 ; e_2dot];

end

== matlab function four_bots_CNN_DSM_7/Multi agent System NN & SMC/Agent 1 /Controller /Estimation ==
  data: phi_x input; W input; E output
function E = estimation(phi_x, W)
%% estimation
E=W'*phi_x;

end

== matlab function four_bots_CNN_DSM_7/Multi agent System NN & SMC/Agent 1 /Controller /Hysteresis/MATLAB Function1 ==
  data: u input; output output; u_dot input; zeta input; zeta_dot output
function [output,zeta_dot] = B_W_hysteresis(u, u_dot, zeta)

mu_1=1.5;
mu_2=3;
beta=1;
chi=0.5;
n=2;

output=mu_1*u+mu_2*zeta;

f=ones(3,1)-beta*sign(u_dot).*abs(zeta).^(n-1).*zeta-chi*abs(zeta).^n;

zeta_dot=u_dot.*f;
end

== matlab function four_bots_CNN_DSM_7/Multi agent System NN & SMC/Agent 1 /Controller /Hysteresis/MATLAB Function2 ==
  data: u input; output output; u_dot input; zeta_1 input; zeta1_dot output
function [output,zeta1_dot] = inv_B_W_hysteresis(u, u_dot, zeta_1)

mu_1=1.5;
mu_2=3;
beta=1;
chi=0.5;
n=2;

output=1/mu_1*u - mu_2/mu_1*zeta_1;

f=ones(3,1)-beta*sign(u_dot/mu_1).*abs(zeta_1).^(n-1).*zeta_1-chi*abs(zeta_1).^n;

zeta1_dot=u_dot.*f./(mu_1+mu_2*f);
end

== matlab function four_bots_CNN_DSM_7/Multi agent System NN & SMC/Agent 2/Controller /Hysteresis/MATLAB Function1 ==
  data: u input; output output; u_dot input; zeta input; zeta_dot output
function [output,zeta_dot] = B_W_hysteresis(u, u_dot, zeta)

mu_1=1.5;
mu_2=3;
beta=1;
chi=0.5;
n=2;

output=mu_1*u+mu_2*zeta;

f=ones(3,1)-beta*sign(u_dot).*abs(zeta).^(n-1).*zeta-chi*abs(zeta).^n;

zeta_dot=u_dot.*f;
end

== matlab function four_bots_CNN_DSM_7/Multi agent System NN & SMC/Agent 2/Controller /Hysteresis/MATLAB Function2 ==
  data: u input; output output; u_dot input; zeta_1 input; zeta1_dot output
function [output,zeta1_dot] = inv_B_W_hysteresis(u, u_dot, zeta_1)

mu_1=1.5;
mu_2=3;
beta=1;
chi=0.5;
n=2;

output=1/mu_1*u - mu_2/mu_1*zeta_1;

f=ones(3,1)-beta*sign(u_dot/mu_1).*abs(zeta_1).^(n-1).*zeta_1-chi*abs(zeta_1).^n;

zeta1_dot=u_dot.*f./(mu_1+mu_2*f);
end

== matlab function four_bots_CNN_DSM_7/Multi agent System NN & SMC/Agent 1 /Controller /Control dot ==
  data: L input; E input; xi input; error input; u_dot output; reference input; u input
function u_dot = control_dot(L, E, xi, error, reference, u)

%% parameters that may change
dimension=3;
c=2.5;
lambda=2.5;
eta=80;
serial_num=1;

num_agent=size(L,1); 
%% codes
r_acc=reference(dimension*num_agent*2+1 : dimension*num_agent*3);
r_accdot=reference(dimension*num_agent*3+1 : dimension*num_agent*4);

xd2_dot = r_acc(dimension*(serial_num-1)+1 : dimension*serial_num);
xd2_ddot = r_accdot(dimension*(serial_num-1)+1 : dimension*serial_num);

e2=error(dimension*1+1:dimension*2);

u_dot= -E + xd2_ddot + (c+lambda)*xd2_dot - (c+lambda)*u -c*lambda*e2 - eta*xi;

end

== matlab function four_bots_CNN_DSM_7/Multi agent System NN & SMC/Agent 2/Controller /Chebyshev Polynomials ==
  data: current_states input; phi_x output
function phi_x = Chebyshev_polynomials(current_states)

%% parameters that may alter
dimension=3;
cheby_order=3;

%% current states
x1=current_states(dimension*0+1:dimension*1);
x2=current_states(dimension*1+1:dimension*2);

%% initialization
phi_x=ones(1+2*dimension*cheby_order,1);

%% recursion procedure
now_x=[x1;x2];
for order = 1 : cheby_order
   if order == 1
      phi_x(2*dimension*(order-1)+2:2*dimension*order+1)=now_x;
   elseif order == 2
      phi_x(2*dimension*(order-1)+2:2*dimension*order+1)=2*now_x.*phi_x(2*dimension*(order-2)+2:2*dimension*(order-1)+1)-1;
   else
      phi_x(2*dimension*(order-1)+2:2*dimension*order+1)=2*now_x.*phi_x(2*dimension*(order-2)+2:2*dimension*(order-1)+1)-phi_x(2*dimension*(order-3)+2:2*dimension*(order-2)+1);
   end
end

end

== matlab function four_bots_CNN_DSM_7/Multi agent System NN & SMC/Agent 2/Controller /Control dot ==
  data: L input; E input; xi input; error input; u_dot output; reference input; u input
function u_dot = control_dot(L, E, xi, error, reference, u)

%% parameters that may change
dimension=3;
c=2.5;
lambda=2.5;
eta=80;

serial_num=2;

num_agent=size(L,1); 
%% codes
r_acc=reference(dimension*num_agent*2+1 : dimension*num_agent*3);
r_accdot=reference(dimension*num_agent*3+1 : dimension*num_agent*4);

xd2_dot = r_acc(dimension*(serial_num-1)+1 : dimension*serial_num);
xd2_ddot = r_accdot(dimension*(serial_num-1)+1 : dimension*serial_num);

e2=error(dimension*1+1:dimension*2);

u_dot= -E + xd2_ddot + (c+lambda)*xd2_dot - (c+lambda)*u -c*lambda*e2 - eta*xi;

end

== matlab function four_bots_CNN_DSM_7/Multi agent System NN & SMC/Agent 1 /Controller /Parameter Tuning ==
  data: phi_x input; xi input; W_dot output
function W_dot = parameter_tuning(phi_x, xi)

%% parameters that may alter
dimension=3;
cheby_order=3;
F=0.1*eye(1+2*dimension*cheby_order);

%% codes
W_dot = F*phi_x*xi';

end

== matlab function four_bots_CNN_DSM_7/Multi agent System NN & SMC/Agent 1 /Controller /Sliding Variable Generation ==
  data: error input; xi output
function xi = sliding_variable(error)

%% parameters that may alter
dimension=3;
c=2.5;
lambda=2.5;

%% codes
error_1=error(dimension*0+1:dimension*1);
error_2=error(dimension*1+1:dimension*2);
error_2dot=error(dimension*2+1:dimension*3);

xi = error_2dot + (c + lambda)* error_2 + lambda * c * error_1;

end

== matlab function four_bots_CNN_DSM_7/Multi agent System NN & SMC/Agent 1 /Controller /neural_initial ==
  data: weight output
function weight = neural_initialize()

% cheby_order   : order of chebyshev polynomials
% dimension     : dimension of the system

cheby_order=3;
dimension=3;

weight = zeros(1+2*cheby_order*dimension, dimension);

end

== matlab function four_bots_CNN_DSM_7/Multi agent System NN & SMC/Agent 2/Controller /Error Calculation ==
  data: cur_states output; current_states input; L input; error output; reference input
function [cur_states , error] = error_calculation(current_states, L, reference)

%% parameters that may change for alternative use
dimension=3;
serial_num=2;

num_agent=size(L,1);
%% current states
% get current states
pos=current_states(dimension*num_agent*0+1 : dimension*num_agent*1);
vol=current_states(dimension*num_agent*1+1 : dimension*num_agent*2);
acc=current_states(dimension*num_agent*2+1 : dimension*num_agent*3);

% get current reference
r_pos=reference(dimension*num_agent*0+1 : dimension*num_agent*1);
r_vol=reference(dimension*num_agent*1+1 : dimension*num_agent*2);
r_acc=reference(dimension*num_agent*2+1 : dimension*num_agent*3);

% agent j's states
agent_x1 = pos(dimension*(serial_num-1)+1 : dimension*serial_num);
agent_x2 = vol(dimension*(serial_num-1)+1 : dimension*serial_num);

% agent_x2dot = acc(dimension*(serial_num-1)+1 : dimension*serial_num);
% 
% % agent j's reference
% r_x1=r_pos(dimension*(serial_num-1)+1 : dimension*serial_num);
% r_x2=r_vol(dimension*(serial_num-1)+1 : dimension*serial_num);
% r_x2dot=r_acc(dimension*(serial_num-1)+1 : dimension*serial_num);

e_1 = kron(L(serial_num, : ), eye(dimension) ) * (pos - r_pos);
e_2 = kron(L(serial_num, : ), eye(dimension) ) * (vol - r_vol);
e_2dot = kron(L(serial_num, : ), eye(dimension) ) * (acc - r_acc);

cur_states = [agent_x1;agent_x2];
error = [e_1 ; e_2 ; e_2dot];

end

== matlab function four_bots_CNN_DSM_7/Multi agent System NN & SMC/Agent 2/Controller /Estimation ==
  data: phi_x input; W input; E output
function E = estimation(phi_x, W)
%% estimation
E=W'*phi_x;

end

== matlab function four_bots_CNN_DSM_7/Multi agent System NN & SMC/Agent 2/Controller /Parameter Tuning ==
  data: phi_x input; xi input; W_dot output
function W_dot = parameter_tuning(phi_x, xi)

%% parameters that may alter
dimension=3;
cheby_order=3;
F=0.1*eye(1+2*dimension*cheby_order);

%% codes
W_dot = F*phi_x*xi';

end

== matlab function four_bots_CNN_DSM_7/Multi agent System NN & SMC/Agent 2/Controller /Sliding Variable Generation ==
  data: error input; xi output
function xi = sliding_variable(error)

%% parameters that may alter
dimension=3;
c=2.5;
lambda=2.5;

%% codes
error_1=error(dimension*0+1:dimension*1);
error_2=error(dimension*1+1:dimension*2);
error_2dot=error(dimension*2+1:dimension*3);

xi = error_2dot + (c + lambda)* error_2 + lambda * c * error_1;

end

== matlab function four_bots_CNN_DSM_7/Multi agent System NN & SMC/Agent 2/Controller /neural_initial ==
  data: weight output
function weight = neural_initialize()

% cheby_order   : order of chebyshev polynomials
% dimension     : dimension of the system

cheby_order=3;
dimension=3;

weight = zeros(1+2*cheby_order*dimension, dimension);

end

== matlab function four_bots_CNN_DSM_7/Multi agent System NN & SMC/Agent 2/MATLAB Function ==
  data: agent_x1 input; x2_dot output; agent_x2 input; t input; control_input input; fx_dt output
function [x2_dot, fx_dt] = physical_model( agent_x1 , agent_x2, t, control_input )

Mass=[4,5,4,5];
Alpha=[0.087,0.090,0.085,0.092];
Radius=[0.18,0.20,0.24,0.22];
Inertia=[0.12,0.15,0.13,0.14];
Beta=[11.4,11.6,11.8,12.0];

%% assign the parameter according to serial number
serial_num = 2; 

m=Mass(serial_num);
alpha=Alpha(serial_num);
R=Radius(serial_num);
inertia=Inertia(serial_num);
beta=Beta(serial_num);

%% current states of the robot
dimension=3;

theta=agent_x1(dimension);

%% the real model of robot
M=diag([1/m,1/m,1/inertia]);
T=[-sin(theta), -sin(pi/3-theta), sin(pi/3+theta);
    cos(theta), -cos(pi/3-theta), -cos(pi/3+theta);
    R,          R,                  R];
uncertain = [0.3*sin(0.5*t)+2; 0.2*cos(0.5*t)+1.5; 0.1*sin(0.3*t)+1];
real_fx = -beta*M*(T*T')*agent_x2;

%% saturation is added here for convinience
Vmax=6; % the maximum voltage of the motor

u1up=Vmax/(alpha*m)*(abs(sin(theta))+abs(sin(pi/3-theta))+abs(sin(pi/3+theta)));
u1do=-Vmax/(alpha*m)*(abs(sin(theta))+abs(sin(pi/3-theta))+abs(sin(pi/3+theta)));
u2up=Vmax/(alpha*m)*(abs(cos(theta))+abs(cos(pi/3-theta))+abs(cos(pi/3+theta)));
u2do=-Vmax/(alpha*m)*(abs(cos(theta))+abs(cos(pi/3-theta))+abs(cos(pi/3+theta)));
u3up=R/(alpha*inertia)*3*Vmax;
u3do=-R/(alpha*inertia)*3*Vmax;

control_input(1) = max( min(control_input(1),u1up), u1do );
control_input(2) = max( min(control_input(2),u2up), u2do );
control_input(3) = max( min(control_input(3),u3up), u3do );




fx_dt= real_fx + uncertain; 
x2_dot = real_fx + control_input + uncertain;


end

== matlab function four_bots_CNN_DSM_7/Multi agent System NN & SMC/Agent 1 /MATLAB Function1 ==
  data: fx_dt input; esti_error output; fx_dtdot input; E input
function esti_error = estimation_error(fx_dt, fx_dtdot, E)

c=2.5;
lambda=2.5;

esti_error = fx_dtdot + (c + lambda) * fx_dt - E; 

end

== matlab function four_bots_CNN_DSM_7/Multi agent System NN & SMC/Agent 2/MATLAB Function1 ==
  data: fx_dt input; esti_error output; fx_dtdot input; E input
function esti_error = estimation_error(fx_dt, fx_dtdot, E)

c=2.5;
lambda=2.5;

esti_error = fx_dtdot + (c + lambda) * fx_dt - E; 

end

== matlab function four_bots_CNN_DSM_7/Multi agent System NN & SMC/Agent 3/Controller /Chebyshev Polynomials ==
  data: current_states input; phi_x output
function phi_x = Chebyshev_polynomials(current_states)

%% parameters that may alter
dimension=3;
cheby_order=3;

%% current states
x1=current_states(dimension*0+1:dimension*1);
x2=current_states(dimension*1+1:dimension*2);

%% initialization
phi_x=ones(1+2*dimension*cheby_order,1);

%% recursion procedure
now_x=[x1;x2];
for order = 1 : cheby_order
   if order == 1
      phi_x(2*dimension*(order-1)+2:2*dimension*order+1)=now_x;
   elseif order == 2
      phi_x(2*dimension*(order-1)+2:2*dimension*order+1)=2*now_x.*phi_x(2*dimension*(order-2)+2:2*dimension*(order-1)+1)-1;
   else
      phi_x(2*dimension*(order-1)+2:2*dimension*order+1)=2*now_x.*phi_x(2*dimension*(order-2)+2:2*dimension*(order-1)+1)-phi_x(2*dimension*(order-3)+2:2*dimension*(order-2)+1);
   end
end

end

== matlab function four_bots_CNN_DSM_7/Multi agent System NN & SMC/Agent 3/Controller /Control dot ==
  data: L input; E input; xi input; error input; u_dot output; reference input; u input
function u_dot = control_dot(L, E, xi, error, reference, u)

%% parameters that may change
dimension=3;
c=2.5;
lambda=2.5;
eta=80;

serial_num=3;

num_agent=size(L,1); 
%% codes
r_acc=reference(dimension*num_agent*2+1 : dimension*num_agent*3);
r_accdot=reference(dimension*num_agent*3+1 : dimension*num_agent*4);

xd2_dot = r_acc(dimension*(serial_num-1)+1 : dimension*serial_num);
xd2_ddot = r_accdot(dimension*(serial_num-1)+1 : dimension*serial_num);

e2=error(dimension*1+1:dimension*2);

u_dot= -E + xd2_ddot + (c+lambda)*xd2_dot - (c+lambda)*u -c*lambda*e2 - eta*xi;

end

== matlab function four_bots_CNN_DSM_7/Multi agent System NN & SMC/Agent 3/Controller /Error Calculation ==
  data: cur_states output; current_states input; L input; error output; reference input
function [cur_states , error] = error_calculation(current_states, L, reference)

%% parameters that may change for alternative use
dimension=3;
serial_num=3;

num_agent=size(L,1);
%% current states
% get current states
pos=current_states(dimension*num_agent*0+1 : dimension*num_agent*1);
vol=current_states(dimension*num_agent*1+1 : dimension*num_agent*2);
acc=current_states(dimension*num_agent*2+1 : dimension*num_agent*3);

% get current reference
r_pos=reference(dimension*num_agent*0+1 : dimension*num_agent*1);
r_vol=reference(dimension*num_agent*1+1 : dimension*num_agent*2);
r_acc=reference(dimension*num_agent*2+1 : dimension*num_agent*3);

% agent j's states
agent_x1 = pos(dimension*(serial_num-1)+1 : dimension*serial_num);
agent_x2 = vol(dimension*(serial_num-1)+1 : dimension*serial_num);

% agent_x2dot = acc(dimension*(serial_num-1)+1 : dimension*serial_num);
% 
% % agent j's reference
% r_x1=r_pos(dimension*(serial_num-1)+1 : dimension*serial_num);
% r_x2=r_vol(dimension*(serial_num-1)+1 : dimension*serial_num);
% r_x2dot=r_acc(dimension*(serial_num-1)+1 : dimension*serial_num);

e_1 = kron(L(serial_num, : ), eye(dimension) ) * (pos - r_pos);
e_2 = kron(L(serial_num, : ), eye(dimension) ) * (vol - r_vol);
e_2dot = kron(L(serial_num, : ), eye(dimension) ) * (acc - r_acc);

cur_states = [agent_x1;agent_x2];
error = [e_1 ; e_2 ; e_2dot];

end

== matlab function four_bots_CNN_DSM_7/Multi agent System NN & SMC/Agent 3/Controller /Estimation ==
  data: phi_x input; W input; E output
function E = estimation(phi_x, W)
%% estimation
E=W'*phi_x;

end

== matlab function four_bots_CNN_DSM_7/Multi agent System NN & SMC/Agent 3/Controller /Parameter Tuning ==
  data: phi_x input; xi input; W_dot output
function W_dot = parameter_tuning(phi_x, xi)

%% parameters that may alter
dimension=3;
cheby_order=3;
F=0.1*eye(1+2*dimension*cheby_order);

%% codes
W_dot = F*phi_x*xi';

end

== matlab function four_bots_CNN_DSM_7/Multi agent System NN & SMC/Agent 3/Controller /Sliding Variable Generation ==
  data: error input; xi output
function xi = sliding_variable(error)

%% parameters that may alter
dimension=3;
c=2.5;
lambda=2.5;

%% codes
error_1=error(dimension*0+1:dimension*1);
error_2=error(dimension*1+1:dimension*2);
error_2dot=error(dimension*2+1:dimension*3);

xi = error_2dot + (c + lambda)* error_2 + lambda * c * error_1;

end

== matlab function four_bots_CNN_DSM_7/Multi agent System NN & SMC/Agent 3/Controller /neural_initial ==
  data: weight output
function weight = neural_initialize()

% cheby_order   : order of chebyshev polynomials
% dimension     : dimension of the system

cheby_order=3;
dimension=3;

weight = zeros(1+2*cheby_order*dimension, dimension);

end
